simulink model "SingleJoint_PID_Considering_Saturation_Block"  (R2023a)
settings: Solver=VariableStepAuto  StartTime=0.0  StopTime=100  RelTol=1e-3  EnableMultiTasking=on
settings Model: Creator=wfxu  LastModifiedBy=17634948724
settings SolverCC: AlgebraicLoopSolver=TrustRegion
settings DataIOCC: LimitDataPoints=on  ReturnWorkspaceOutputs=off
settings OptimizationCC: LifeSpan=inf
settings DebuggingCC: UnconnectedInputMsg=warning  UnconnectedOutputMsg=warning  UnconnectedLineMsg=warning  AllowSymbolicDim=off  SFUnexpectedBacktrackingDiag=warning  SFNoUnconditionalDefaultTransitionDiag=warning  SFExecutionAtInitializationDiag=none  ArithmeticOperatorsInVariantConditions=warning
settings ModelReferenceCC: EnableRefExpFcnMdlSchedulingChecks=on  PropagateSignalLabelsOutOfModel=off
settings SFSimCC: SimUseLocalCustomCode=off  CustomCodeUndefinedFunction=UseInterfaceOnly
settings RTWCC: RTWUseLocalCustomCode=off
settings CodeAppCC: StateflowObjectComments=on
settings GRTTargetCC: TargetLangStandard=C89/C90 (ANSI)
settings ConfigComp: CovMetricSettings=dw  CovSaveCumulativeToWorkspaceVar=on  CovSaveSingleToWorkspaceVar=on  CovExternalEMLEnable=off

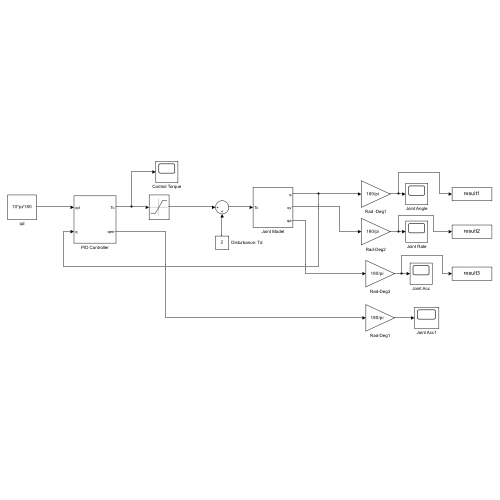
[thumbnail: Simulink's stored preview of the top-level diagram]
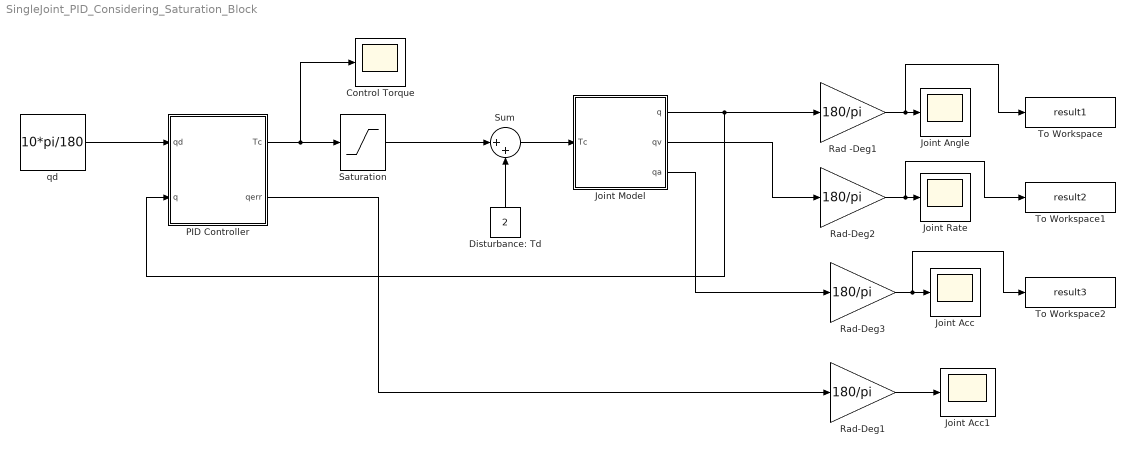
== system SingleJoint_PID_Considering_Saturation_Block ==
  Control Torque : Scope
  Disturbance: Td : Constant  Value=2
  Joint Acc : Scope
  Joint Acc1 : Scope
  Joint Angle : Scope
  Joint Model : Subsystem
  Joint Rate : Scope
  "PID Controller " : Subsystem
  Rad -Deg1 : Gain  Gain=180/pi
  Rad-Deg1 : Gain  Gain=180/pi
  Rad-Deg2 : Gain  Gain=180/pi
  Rad-Deg3 : Gain  Gain=180/pi
  Saturation : Saturate  UpperLimit=20  LowerLimit=-20  ZeroCross=off
  Sum : Sum  Inputs=|++
  To Workspace : ToWorkspace  VariableName=result1  SaveFormat=Timeseries  SampleTime=-1
  To Workspace1 : ToWorkspace  VariableName=result2  SaveFormat=Timeseries  SampleTime=-1
  To Workspace2 : ToWorkspace  VariableName=result3  SaveFormat=Timeseries  SampleTime=-1
  qd : Constant  Value=10*pi/180
  wires:
  "PID Controller "/1(Tc) -> Control Torque/1, Saturation/1
  Joint Model/1(q) -> Rad -Deg1/1, "PID Controller "/2(q)
  qd/1 -> "PID Controller "/1(qd)
  Saturation/1 -> Sum/1
  Disturbance: Td/1 -> Sum/2
  Sum/1 -> Joint Model/1(Tc)
  Rad-Deg3/1 -> To Workspace2/1, Joint Acc/1
  Rad -Deg1/1 -> To Workspace/1, Joint Angle/1
  Rad-Deg2/1 -> To Workspace1/1, Joint Rate/1
  Joint Model/2(qv) -> Rad-Deg2/1
  Joint Model/3(qa) -> Rad-Deg3/1
  Rad-Deg1/1 -> Joint Acc1/1
  "PID Controller "/2(qerr) -> Rad-Deg1/1

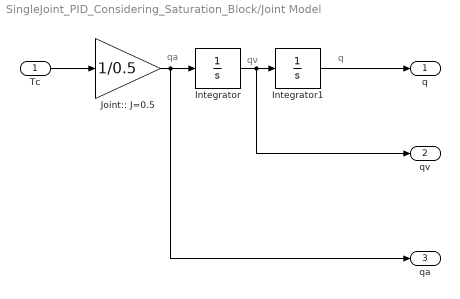
== system SingleJoint_PID_Considering_Saturation_Block/Joint Model ==
  note: qa
  note: qv
  note: q
  Tc : Inport
  Integrator : Integrator
  Integrator1 : Integrator
  Joint:: J=0.5 : Gain  Gain=1/0.5
  q : Outport
  qv : Outport  Port=2
  qa : Outport  Port=3
  wires:
  Integrator1/1 -> q/1
  Integrator/1 -> qv/1, Integrator1/1
  Joint:: J=0.5/1 -> qa/1, Integrator/1
  Tc/1 -> Joint:: J=0.5/1

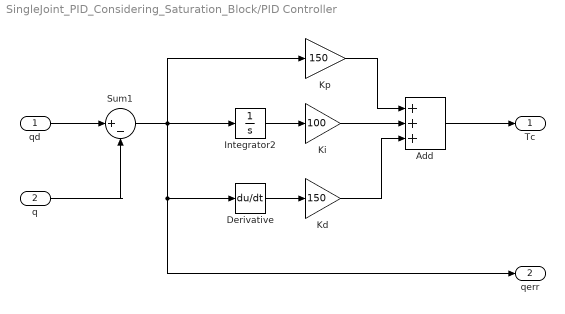
== system SingleJoint_PID_Considering_Saturation_Block/PID Controller  ==
  qd : Inport
  q : Inport  Port=2
  Add : Sum  Inputs=+++
  Derivative : Derivative
  Integrator2 : Integrator
  Kd : Gain  Gain=150
  Ki : Gain  Gain=100
  Kp : Gain  Gain=150
  Sum1 : Sum  Inputs=|+-
  Tc : Outport
  qerr : Outport  Port=2
  wires:
  Kd/1 -> Add/3
  Ki/1 -> Add/2
  Add/1 -> Tc/1
  Integrator2/1 -> Ki/1
  Kp/1 -> Add/1
  Derivative/1 -> Kd/1
  qd/1 -> Sum1/1
  q/1 -> Sum1/2
  Sum1/1 -> qerr/1, Derivative/1, Kp/1, Integrator2/1
